simulink model "Partial_Quadcopter_simulation"  (R2017a)
settings: Solver=ode45  StartTime=0.0  StopTime=2  FixedStep=0.05  MaxStep=0.06  RelTol=1e-3  EnableMultiTasking=on
model workspace (MAT data in the model file):
  MCOS : class17 (value not decoded)
undefined symbols (not defined in the file or in its folder): error1, error2, error3, error4, IC, quadModel
libraries: simulink x4
(part 2 of 2)

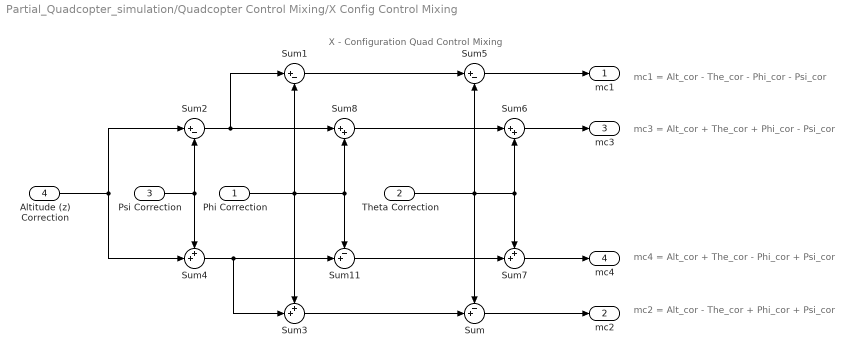
== system Partial_Quadcopter_simulation/Quadcopter Control Mixing/X Config Control Mixing ==
  note: mc1 = Alt_cor - The_cor - Phi_cor - Psi_cor
  note: X - Configuration Quad Control Mixing
  note: mc3 = Alt_cor + The_cor + Phi_cor - Psi_cor
  note: mc2 = Alt_cor - The_cor + Phi_cor + Psi_cor
  note: mc4 = Alt_cor + The_cor - Phi_cor + Psi_cor
  Phi Correction : Inport
  Theta Correction : Inport  Port=2
  Psi Correction : Inport  Port=3
  Altitude (z) Correction : Inport  Port=4
  Sum : Sum  Inputs=-+|
  Sum1 : Sum  Inputs=|+-
  Sum11 : Sum  Inputs=-+|
  Sum2 : Sum  Inputs=|+-
  Sum3 : Sum  Inputs=++|
  Sum4 : Sum  Inputs=++|
  Sum5 : Sum  Inputs=|+-
  Sum6 : Sum  Inputs=|++
  Sum7 : Sum  Inputs=++|
  Sum8 : Sum  Inputs=|++
  mc1 : Outport
  mc2 : Outport  Port=2
  mc3 : Outport  Port=3
  mc4 : Outport  Port=4
  wires:
  Sum2/1 -> Sum8/1, Sum1/1
  Psi Correction/1 -> Sum4/1, Sum2/2
  Phi Correction/1 -> Sum3/1, Sum1/2, Sum8/2, Sum11/1
  Sum4/1 -> Sum3/2, Sum11/2
  Sum3/1 -> Sum/2
  Theta Correction/1 -> Sum7/1, Sum6/2, Sum5/2, Sum/1
  Sum1/1 -> Sum5/1
  Sum8/1 -> Sum6/1
  Sum11/1 -> Sum7/2
  Sum5/1 -> mc1/1
  Sum6/1 -> mc3/1
  Sum7/1 -> mc4/1
  Altitude (z) Correction/1 -> Sum2/1, Sum4/2
  Sum/1 -> mc2/1

== system Partial_Quadcopter_simulation/Quadcopter Dynamics/External Disturbances ==
  note: Note: Torques are in units of N*m, Forces in N
      | Torques are applied to the BODY coordinate system.
      | Forces are applied from the WORLD coordinate system!
      | This can be changed by adjusting the equations within the S-function.
  Bus Creator : BusCreator  Inputs=6
  Bus to Vector : BusToVector
  Constant{2..6} (5 alike) : Constant  Value=0
  Step : Step  After=0  SampleTime=0
  "Disturbances " : Outport
  wires:
  Bus to Vector/1 -> "Disturbances "/1
  Bus Creator/1 -> Bus to Vector/1
  Constant6/1 -> Bus Creator/1  "Tau_bx-axis"
  Step/1 -> Bus Creator/2  "Tau_by-axis"
  Constant2/1 -> Bus Creator/3  "Tau_bz-axis"
  Constant3/1 -> Bus Creator/4  "Force_x-axis"
  Constant4/1 -> Bus Creator/5  "Force_y-axis"
  Constant5/1 -> Bus Creator/6  "Force_z-axis"

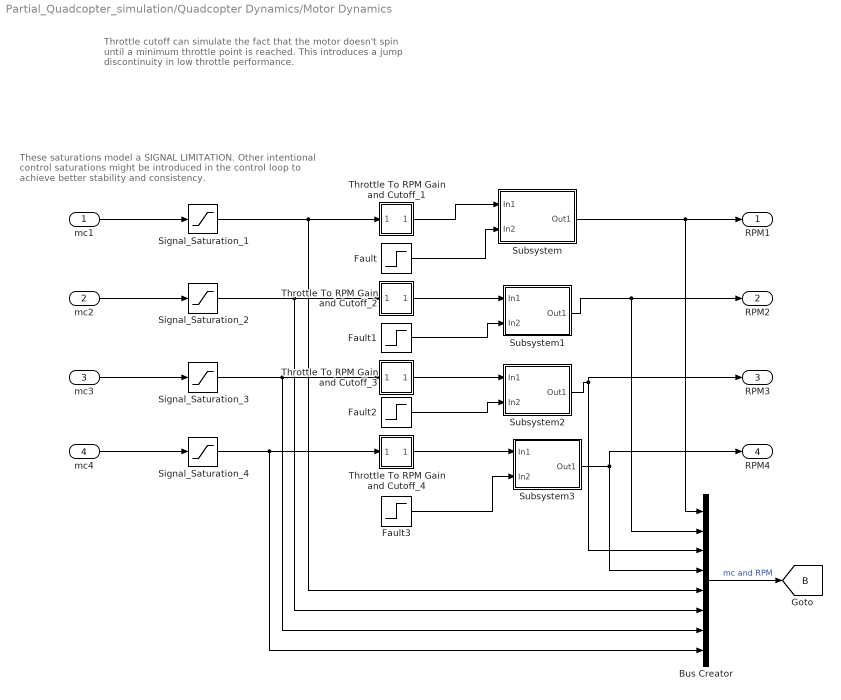
== system Partial_Quadcopter_simulation/Quadcopter Dynamics/Motor Dynamics ==
  note: Throttle cutoff can simulate the fact that the motor doesn't
      | spin until a minimum throttle point is reached. This introduces
      | a jump discontinuity in low throttle performance.
  note: These saturations model a SIGNAL LIMITATION.
      | Other intentional control saturations might be introduced in the
      | control loop to achieve better stability and consistency.
  mc1 : Inport
  mc2 : Inport  Port=2
  mc3 : Inport  Port=3
  mc4 : Inport  Port=4
  Bus Creator : BusCreator  Inputs=8
  Fault : Step  Time=0  After=error1  SampleTime=0
  Fault1 : Step  Time=0  After=error2  SampleTime=0
  Fault2 : Step  Time=0  After=error3  SampleTime=0
  Fault3 : Step  Time=0  After=error4  SampleTime=0
  Signal_Saturation_{1..4} (4 alike) : Saturate  UpperLimit=100  LowerLimit=0
  Subsystem : Subsystem
  Subsystem1 : Subsystem
  Subsystem2 : Subsystem
  Subsystem3 : Subsystem
  Throttle To RPM Gain and Cutoff_1 : Subsystem
  Throttle To RPM Gain and Cutoff_2 : Subsystem
  Throttle To RPM Gain and Cutoff_3 : Subsystem
  Throttle To RPM Gain and Cutoff_4 : Subsystem
  RPM1 : Outport
  RPM2 : Outport  Port=2
  RPM3 : Outport  Port=3
  RPM4 : Outport  Port=4
  tag scope: B=global
  wires:
  mc1/1 -> Signal_Saturation_1/1
  mc4/1 -> Signal_Saturation_4/1
  mc2/1 -> Signal_Saturation_2/1
  mc3/1 -> Signal_Saturation_3/1
  Signal_Saturation_1/1 -> Bus Creator/5, Throttle To RPM Gain and Cutoff_1/1(In5)
  Signal_Saturation_2/1 -> Bus Creator/6, Throttle To RPM Gain and Cutoff_2/1(In5)
  Signal_Saturation_3/1 -> Bus Creator/7, Throttle To RPM Gain and Cutoff_3/1(In5)
  Signal_Saturation_4/1 -> Bus Creator/8, Throttle To RPM Gain and Cutoff_4/1(In5)
  Throttle To RPM Gain and Cutoff_4/1(Out5) -> Subsystem3/1(In1)
  Subsystem3/1(Out1) -> RPM4/1, Bus Creator/4
  Bus Creator/1 -> [B]  "mc and RPM"
  Subsystem/1(Out1) -> Bus Creator/1, RPM1/1
  Throttle To RPM Gain and Cutoff_1/1(Out5) -> Subsystem/1(In1)
  Fault/1 -> Subsystem/2(In2)
  Subsystem2/1(Out1) -> Bus Creator/3, RPM3/1
  Subsystem1/1(Out1) -> Bus Creator/2, RPM2/1
  Throttle To RPM Gain and Cutoff_2/1(Out5) -> Subsystem1/1(In1)
  Throttle To RPM Gain and Cutoff_3/1(Out5) -> Subsystem2/1(In1)
  Fault2/1 -> Subsystem2/2(In2)
  Fault3/1 -> Subsystem3/2(In2)
  Fault1/1 -> Subsystem1/2(In2)

== system Partial_Quadcopter_simulation/Quadcopter Dynamics/Motor Dynamics/Subsystem ==
  In1 : Inport
  In2 : Inport  Port=2
  MATLAB Function : MATLAB Function  TreatAsAtomicUnit=on
  Motor_Dynamics_1 : StateSpace  A=-1/quadModel.T  C=1/quadModel.T  D=0  X0=IC.w1*quadModel.T
  Scope : Scope  NumInputPorts=4
  Out1 : Outport
  wires:
  In1/1 -> Motor_Dynamics_1/1
  MATLAB Function/1(rotor_speed) -> Scope/3, Out1/1
  In2/1 -> MATLAB Function/1(fault)
  Motor_Dynamics_1/1 -> Scope/2, MATLAB Function/2(nominal_model_input)

== system Partial_Quadcopter_simulation/Quadcopter Dynamics/Motor Dynamics/Subsystem1 ==
  In1 : Inport
  In2 : Inport  Port=2
  MATLAB Function : MATLAB Function  TreatAsAtomicUnit=on
  "Motor_Dynamics_2 " : StateSpace  A=-1/quadModel.T  C=1/quadModel.T  D=0  X0=IC.w1*quadModel.T
  Out1 : Outport
  wires:
  In1/1 -> "Motor_Dynamics_2 "/1
  MATLAB Function/1(rotor_speed) -> Out1/1
  In2/1 -> MATLAB Function/1(fault)
  "Motor_Dynamics_2 "/1 -> MATLAB Function/2(nominal_modal_input)

== system Partial_Quadcopter_simulation/Quadcopter Dynamics/Motor Dynamics/Subsystem2 ==
  In1 : Inport
  In2 : Inport  Port=2
  MATLAB Function : MATLAB Function  TreatAsAtomicUnit=on
  "Motor_Dynamics_3 " : StateSpace  A=-1/quadModel.T  C=1/quadModel.T  D=0  X0=IC.w1*quadModel.T
  Out1 : Outport
  wires:
  In1/1 -> "Motor_Dynamics_3 "/1
  MATLAB Function/1(rotor_speed) -> Out1/1
  In2/1 -> MATLAB Function/1(fault)
  "Motor_Dynamics_3 "/1 -> MATLAB Function/2(nominal_modal_input)

== system Partial_Quadcopter_simulation/Quadcopter Dynamics/Motor Dynamics/Subsystem3 ==
  In1 : Inport
  In2 : Inport  Port=2
  MATLAB Function : MATLAB Function  TreatAsAtomicUnit=on
  "Motor_Dynamics_4 " : StateSpace  A=-1/quadModel.T  C=1/quadModel.T  D=0  X0=IC.w1*quadModel.T
  Out1 : Outport
  wires:
  In1/1 -> "Motor_Dynamics_4 "/1
  MATLAB Function/1(rotor_speed) -> Out1/1
  In2/1 -> MATLAB Function/1(fault)
  "Motor_Dynamics_4 "/1 -> MATLAB Function/2(nominal_modal_input)

== system Partial_Quadcopter_simulation/Quadcopter Dynamics/Motor Dynamics/Throttle To RPM Gain and Cutoff_1 ==
  note: minThr should be a quad.mat value
  note: This gain should be a quad.mat value
  note: This constant should be a quad.mat value
  note: Output equals linearly scaled RPM
      | for given throttle input if throttle input >=Throttle Cuttoff (minThr)
      | else output is zero.
  In5 : Inport
  Constant : Constant  Value=quadModel.b
  Gain : Gain  Gain=quadModel.cr
  Minimum Throttle Cutoff : simulink/Logic and Bit Operations/Compare To Constant  relop=>=  const=quadModel.minThr  OutDataTypeStr=uint8
  Product : Product
  Sum1 : Sum  Inputs=++|
  Out5 : Outport
  wires:
  Minimum Throttle Cutoff/1 -> Product/2
  Product/1 -> Out5/1
  In5/1 -> Gain/1, Minimum Throttle Cutoff/1
  Gain/1 -> Sum1/2
  Sum1/1 -> Product/1
  Constant/1 -> Sum1/1

== system Partial_Quadcopter_simulation/Quadcopter Dynamics/Motor Dynamics/Throttle To RPM Gain and Cutoff_2 ==
  note: minThr should be a quad.mat value
  note: This gain should be a quad.mat value
  note: This constant should be a quad.mat value
  note: Output equals linearly scaled RPM
      | for given throttle input if throttle input >=Throttle Cuttoff (minThr)
      | else output is zero.
  In5 : Inport
  Constant : Constant  Value=quadModel.b
  Gain : Gain  Gain=quadModel.cr
  Minimum Throttle Cutoff : simulink/Logic and Bit Operations/Compare To Constant  relop=>=  const=quadModel.minThr  OutDataTypeStr=uint8
  Product : Product
  Sum1 : Sum  Inputs=++|
  Out5 : Outport
  wires:
  Minimum Throttle Cutoff/1 -> Product/2
  Product/1 -> Out5/1
  In5/1 -> Gain/1, Minimum Throttle Cutoff/1
  Gain/1 -> Sum1/2
  Sum1/1 -> Product/1
  Constant/1 -> Sum1/1

== system Partial_Quadcopter_simulation/Quadcopter Dynamics/Motor Dynamics/Throttle To RPM Gain and Cutoff_3 ==
  note: minThr should be a quad.mat value
  note: This gain should be a quad.mat value
  note: This constant should be a quad.mat value
  note: Output equals linearly scaled RPM
      | for given throttle input if throttle input >=Throttle Cuttoff (minThr)
      | else output is zero.
  In5 : Inport
  Constant : Constant  Value=quadModel.b
  Gain : Gain  Gain=quadModel.cr
  Minimum Throttle Cutoff : simulink/Logic and Bit Operations/Compare To Constant  relop=>=  const=quadModel.minThr  OutDataTypeStr=uint8
  Product : Product
  Sum1 : Sum  Inputs=++|
  Out5 : Outport
  wires:
  Minimum Throttle Cutoff/1 -> Product/2
  Product/1 -> Out5/1
  In5/1 -> Gain/1, Minimum Throttle Cutoff/1
  Gain/1 -> Sum1/2
  Sum1/1 -> Product/1
  Constant/1 -> Sum1/1

== system Partial_Quadcopter_simulation/Quadcopter Dynamics/Motor Dynamics/Throttle To RPM Gain and Cutoff_4 ==
  note: minThr should be a quad.mat value
  note: This gain should be a quad.mat value
  note: This constant should be a quad.mat value
  note: Output equals linearly scaled RPM
      | for given throttle input if throttle input >=Throttle Cuttoff (minThr)
      | else output is zero.
  In5 : Inport
  Constant : Constant  Value=quadModel.b
  Gain : Gain  Gain=quadModel.cr
  Minimum Throttle Cutoff : simulink/Logic and Bit Operations/Compare To Constant  relop=>=  const=quadModel.minThr  OutDataTypeStr=uint8
  Product : Product
  Sum1 : Sum  Inputs=++|
  Out5 : Outport
  wires:
  Minimum Throttle Cutoff/1 -> Product/2
  Product/1 -> Out5/1
  In5/1 -> Gain/1, Minimum Throttle Cutoff/1
  Gain/1 -> Sum1/2
  Sum1/1 -> Product/1
  Constant/1 -> Sum1/1

== matlab function Partial_Quadcopter_simulation/Quadcopter Dynamics/Motor Dynamics/Subsystem/MATLAB Function ==
  data: fault input; nominal_model_input input; rotor_speed output
function rotor_speed = fcn(fault, nominal_model_input)

rotor_speed =(nominal_model_input* (1-fault));

end

== matlab function Partial_Quadcopter_simulation/Attitude Controller/blending  ==
  data: control_signal output; portion input; fault_controller input; nominal_controller input
function control_signal = blending(portion , fault_controller, nominal_controller)

fault_part = (fault_controller * portion);
nominal_portion = 1-portion;
nominal_part = nominal_controller * nominal_portion;
control_signal = fault_part + nominal_part;

end

== matlab function Partial_Quadcopter_simulation/Quadcopter Dynamics/Motor Dynamics/Subsystem1/MATLAB Function ==
  data: fault input; nominal_modal_input input; rotor_speed output
function rotor_speed = fcn(  fault, nominal_modal_input)


rotor_speed =  (nominal_modal_input* (1-fault));

end

== matlab function Partial_Quadcopter_simulation/Position Controller/MATLAB Function ==
  data: y_error input; x_error input; sim_error_store data_store_memory
function fcn(y_error,x_error)
global sim_error_store;

%if(abs(y_error) + abs(x_error) > max_error_signal)
sim_error_store = sim_error_store + abs(y_error) + abs(x_error);
end

== matlab function Partial_Quadcopter_simulation/Quadcopter Dynamics/Motor Dynamics/Subsystem2/MATLAB Function ==
  data: fault input; nominal_modal_input input; rotor_speed output
function rotor_speed = fcn(  fault, nominal_modal_input)


rotor_speed =  (nominal_modal_input* (1-fault));

end

== matlab function Partial_Quadcopter_simulation/Quadcopter Dynamics/Motor Dynamics/Subsystem3/MATLAB Function ==
  data: fault input; nominal_modal_input input; rotor_speed output
function rotor_speed = fcn(  fault, nominal_modal_input)


rotor_speed =  (nominal_modal_input* (1-fault));

end

== matlab function Partial_Quadcopter_simulation/Attitude Controller/blending 1 ==
  data: control_signal output; portion input; fault_controller input; nominal_controller input
function control_signal = blending(portion , fault_controller, nominal_controller)

fault_part = (fault_controller * portion);
nominal_portion = 1-portion;
nominal_part = nominal_controller * nominal_portion;
control_signal = fault_part + nominal_part;

end

== matlab function Partial_Quadcopter_simulation/Attitude Controller/blending 2 ==
  data: control_signal output; portion input; fault_controller input; nominal_controller input
function control_signal = blending(portion , fault_controller, nominal_controller)

fault_part = (fault_controller * portion);
nominal_portion = 1-portion;
nominal_part = nominal_controller * nominal_portion;
control_signal = fault_part + nominal_part;

end

== matlab function Partial_Quadcopter_simulation/Subsystem1/MATLAB Function ==
  data: P_in input; Q_in input; R_in input; Phi_in input; The_in input; U_in input; W_in input; X_in input; Y_in input; Psi_in input; P output; Q output; R output; Phi output; The output; U output; W output; V_in input; Z_in input; X output; Y output; Psi output; V output; Z output; rotor_speed1 output; rotor_speed2 output; rotor_speed3 output; rotor_speed4 output; signal_5 output; signal_6 output; signal_7 output; signal_8 output; r1_speed input; r2_speed input; r3_speed input; Attitude_cmd output; XY_Cmd output; r4_speed input; sig_5 input; sig_6 input; sig_8 input; sig_7 input; Phi_Cmd input; The_Cmd input; Psi_Cmd input; Alt_Cmd input; X_Cmd input; Y_Cmd input
function [P, Q , R , Phi , The , U , W , X, Y, Psi, V, Z ,  rotor_speed1, rotor_speed2, rotor_speed3, rotor_speed4, signal_5, signal_6, signal_7, signal_8 , Attitude_cmd, XY_Cmd]  = fcn( P_in, Q_in , R_in , Phi_in , The_in , U_in , W_in , X_in, Y_in, Psi_in, V_in, Z_in ,  r1_speed ,r2_speed,r3_speed,r4_speed, sig_5 , sig_6, sig_8, sig_7 , Phi_Cmd, The_Cmd, Psi_Cmd, Alt_Cmd, X_Cmd, Y_Cmd  )

global sim_iteration ; 
global sim_state;

if(sim_iteration == 0)
    P = sim_state.P;
    Q = sim_state.Q;
    R = sim_state.R;
    Phi = sim_state.Phi;
    The = sim_state.The;
    U = sim_state.U;
    W = sim_state.W;
    X = sim_state.X;
    Y = sim_state.Y;
    Psi = sim_state.Psi;
    V = sim_state.V;
    Z = sim_state.Z;
    rotor_speed1 = sim_state.r1_speed;
    rotor_speed2 = sim_state.r2_speed;
    rotor_speed3 = sim_state.r3_speed;
    rotor_speed4 = sim_state.r4_speed;
    signal_5 = sim_state.sig_5;
    signal_6 = sim_state.sig_6;
    signal_8 = sim_state.sig_8;
    signal_7 = sim_state.sig_7;
    Phi_Cmd = sim_state.Phi_Cmd;
    The_Cmd = sim_state.The_Cmd;
    Psi_Cmd = sim_state.Psi_Cmd;
    Alt_Cmd = sim_state.Alt_Cmd;
    X_Cmd = sim_state.X_Cmd;
    Y_Cmd = sim_stateY_Cmd;

    
else 
    P = P_in;
    Q = Q_in;
    R = R_in;
    Phi = Phi_in;
    The = The_in;
    U = U_in;
    W = W_in;
    X = X_in;
    Y = Y_in;
    Psi = Psi_in;
    V = V_in;
    Z = Z_in;
    mc_rpm = mc_RPM_in;
    Attitude_cmd = Attitude_cmd_in;
    XY_Cmd = XY_Cmd_in;

end
sim_iteration = sim_iteration+1;

== matlab function Partial_Quadcopter_simulation/Subsystem/MATLAB Function2 ==
  data: P output; Q output; R output; Phi output; The output; Psi output; U output; V output; W output; X output; Y output; Z output; rotor_speed1 output; rotor_speed2 output; rotor_speed3 output; rotor_speed4 output; signal_5 output; signal_6 output; signal_7 output; signal_8 output; Phi_cmd output; The_cmd output; Psi_cmd output; Alt_Cmd output; X_cmd output; Y_cmd output; sim_state_X data_store_memory; sim_state_Y data_store_memory; sim_state_Z data_store_memory; sim_state_U data_store_memory; sim_state_V data_store_memory; sim_state_W data_store_memory; sim_state_Psi data_store_memory; sim_state_P data_store_memory; sim_state_Q data_store_memory; sim_state_R data_store_memory; sim_state_Phi data_store_memory; sim_state_The data_store_memory; sim_state_r1_speed data_store_memory; sim_state_r2_speed data_store_memory; sim_state_r3_speed data_store_memory; sim_state_r4_speed data_store_memory; sim_state_sig_5 data_store_memory; sim_state_sig_6 data_store_memory; sim_state_sig_7 data_store_memory; sim_state_sig_8 data_store_memory; sim_state_Phi_Cmd data_store_memory; sim_state_The_Cmd data_store_memory; sim_state_Psi_Cmd data_store_memory; sim_state_Alt_Cmd data_store_memory; sim_state_X_Cmd data_store_memory; sim_state_Y_Cmd data_store_memory; error1 data_store_memory; error2 data_store_memory; error3 data_store_memory; error4 data_store_memory; Phi_sim_blend data_store_memory; Theta_sim_blend data_store_memory; Psi_sim_blend data_store_memory; sim_iteration data_store_memory
function [P, Q , R , Phi , The ,Psi, U , V,W , X, Y,Z ,  rotor_speed1, rotor_speed2, rotor_speed3, rotor_speed4, signal_5, signal_6, signal_7, signal_8 , Phi_cmd,  The_cmd , Psi_cmd ,   Alt_Cmd ,X_cmd ,Y_cmd ]  = fcn

global sim_iteration;
global sim_state_P;
global sim_state_Q;
global sim_state_R;
global sim_state_Phi;
global sim_state_The;
global sim_state_Psi;
global sim_state_U;
global sim_state_V;
global sim_state_W;
global sim_state_X;
global sim_state_Y;
global sim_state_Z;
global sim_state_r1_speed;
global sim_state_r2_speed;
global sim_state_r3_speed;
global sim_state_r4_speed;
global sim_state_sig_5;
global sim_state_sig_6;
global sim_state_sig_7;
global sim_state_sig_8;
global sim_state_Phi_Cmd;
global sim_state_The_Cmd;
global sim_state_Psi_Cmd;
global sim_state_Alt_Cmd;
global sim_state_X_Cmd;
global sim_state_Y_Cmd;


    P = sim_state_P;
    Q = sim_state_Q;
    R = sim_state_R;
    Phi = sim_state_Phi;
    The = sim_state_The;
    U = sim_state_U;
    W = sim_state_W;
    X = sim_state_X;
    Y = sim_state_Y;
    Psi = sim_state_Psi;
    V = sim_state_V;
    Z = sim_state_Z;
    rotor_speed1 = sim_state_r1_speed;
    rotor_speed2 = sim_state_r2_speed;
    rotor_speed3 = sim_state_r3_speed;
    rotor_speed4 = sim_state_r4_speed;
    signal_5 = sim_state_sig_5;
    signal_6 = sim_state_sig_6;
    signal_8 = sim_state_sig_8;
    signal_7 = sim_state_sig_7;
    Phi_cmd = sim_state_Phi_Cmd;
    The_cmd = sim_state_The_Cmd;
    Psi_cmd = sim_state_Psi_Cmd;
    Alt_Cmd = sim_state_Alt_Cmd;
    X_cmd = sim_state_X_Cmd;
    Y_cmd = sim_state_Y_Cmd;
